simulink model "pmsm"  (R2021a)
settings: Solver=VariableStepAuto  StartTime=0.0  StopTime=5  RelTol=1e-3
values from neighbouring files (symbols this model uses):
  Fr = 5e-5    (= 5e-05)    [parame.m]
  J = 1.1e-3    (= 0.0011)    [parame.m]
  Ld = 1.8e-3    (= 0.0018)    [parame.m]
  Lq = 1.8e-3    (= 0.0018)    [parame.m]
  P = 2    [parame.m]
  Qf = 0.14    [parame.m]
  Rs = 0.76    [parame.m]
  Tmli = 1/fmli    (= 0.000333333333333)    [parame.m]
  Vdc = 220    [parame.m]
undefined symbols (not defined in the file or in its folder): sigbuilder_block
libraries: spsIGBTDiodeLib x6, spsVoltageMeasurementLib x3, spsDCVoltageSourceLib x1, simulink x1, spspowerguiLib x1
settings Model: Creator=21277  LastModifiedBy=PRO
settings SolverCC: AlgebraicLoopSolver=TrustRegion
settings OptimizationCC: LifeSpan=inf
settings DebuggingCC: UnconnectedInputMsg=none  UnconnectedOutputMsg=none  UnconnectedLineMsg=none  SFMachineParentedDataDiag=warning  ArithmeticOperatorsInVariantConditions=warning
settings ModelReferenceCC: EnableRefExpFcnMdlSchedulingChecks=off
settings SFSimCC: CustomCodeUndefinedFunction=UseInterfaceOnly
settings RTWCC: Description=Generic Real-Time Target
settings CodeAppCC: StateflowObjectComments=on

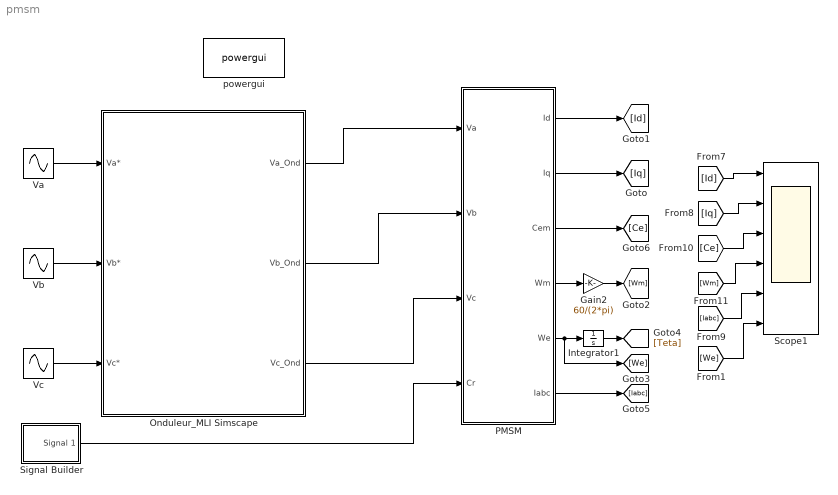
== system pmsm ==
  Gain2 : Gain  Gain=60/(2*pi)
  Integrator1 : Integrator
  Onduleur_MLI Simscape : Subsystem
  PMSM : Subsystem
  Scope1 : Scope  NumInputPorts=6
  Signal Builder : Subsystem  Tag=STV Subsys  LoadFcn=sigbuilder_block('load');  StartFcn=sigbuilder_block('start');  StopFcn=sigbuilder_block('stop');  ClipboardFcn=sigbuilder_block('clipboard');  mask(Sigbuilder block){tuvar=[0:10]}
      mask help: Simulink:masks:SigbuilderBlock_MD
      mask init:
      | if ~strcmp(get_param(bdroot(gcbh),'SimulationStatus'),'stopped') tuvar = sigbuilder_block('maskInit'); end
      settings: CopyFcn=sigbuilder_block('copy');  DeleteFcn=sigbuilder_block('delete');  ModelCloseFcn=sigbuilder_block('modelClose');  PreSaveFcn=sigbuilder_block('preSave');  PauseFcn=sigbuilder_block('pause');  ContinueFcn=sigbuilder_block('continue');  NameChangeFcn=sigbuilder_block('namechange');  OpenFcn=sigbuilder_block('open',[442.8 160.8 550.8 400.2 ]);  CloseFcn=sigbuilder_block('close');
      mask Display: plot(0, 0, 100, 100,[2, 2, 32, 32, 2], [68, 8, 8, 68, 68],[32, 2], [38, 38], [32, 19, 2],[53, 60, 44], [32, 17, 17, 2],[16, 16, 31, 31]);txt = getActiveGroup(gcbh);text(2, 100, txt,'verticalAlignment', 'top');
  Va : Sin  Amplitude=100  Frequency=50  SampleTime=0
  Vb : Sin  Amplitude=100  Frequency=50  Phase=-2*pi/3  SampleTime=0
  Vc : Sin  Amplitude=100  Frequency=50  Phase=2*pi/3  SampleTime=0
  powergui : spspowerguiLib/powergui  Priority=1  SimulationMode=Discrete  SampleTime=1e-5  frequency=60  Iterations=50  frequencyindice=0  Pbase=100e6  ErrMax=1e-4  UnitsV=kV  UnitsW=MW  buscounter=0  FunctionMessages=off  echomessages=off  EnableUseOfTLC=off  CurrentSourceSwitches=off  DisableSnubberDevices=off  DisableRonSwitches=off  DisableVfSwitches=off  DisplayEquations=off  AutomaticDiscreteSolvers=off  SolverType=Tustin/Backward Euler (TBE)  Interpol=off  ExternalGateDelay=off  methode=off  Ts=100  x0status=blocks  SPID=on  SwTol=0  HookPort=off  NonlinearTolerance=1e-4  nMaxIteration=100  ContinueOnMaxIteration=off  RestoreLinks=warning  ResistiveCurrentMeasurement=off  Frange=[0:2:500]  Ylog=off  Xlog=on  ShowGrid=off  save=off  variable=ZData  structure=0  ZoomFFT=off  StartTime=0.0  cycles=1  DisplayStyle=1  fundamental=60  FreqAxis=off  MaxFrequency=1000  frequencyindicesteady=1  RmsSteady=1  display=off
  wires:
  [Iabc] -> Scope1/5
  Signal Builder/1(Signal 1) -> PMSM/4(Cr)
  PMSM/6(Iabc) -> [Iabc]
  [Id] -> Scope1/1
  Gain2/1 -> [Wm]
  [Ce] -> Scope1/3
  [Iq] -> Scope1/2
  PMSM/1(Id) -> [Id]
  Onduleur_MLI Simscape/2(Vb_Ond) -> PMSM/2(Vb)
  [Wm] -> Scope1/4
  PMSM/5(We) -> Integrator1/1, [We]
  PMSM/2(Iq) -> [Iq]
  PMSM/4(Wm) -> Gain2/1
  Onduleur_MLI Simscape/3(Vc_Ond) -> PMSM/3(Vc)
  PMSM/3(Cem) -> [Ce]
  Onduleur_MLI Simscape/1(Va_Ond) -> PMSM/1(Va)
  Integrator1/1 -> [Teta]
  [We] -> Scope1/6
  Va/1 -> Onduleur_MLI Simscape/1(Va*)
  Vb/1 -> Onduleur_MLI Simscape/2(Vb*)
  Vc/1 -> Onduleur_MLI Simscape/3(Vc*)

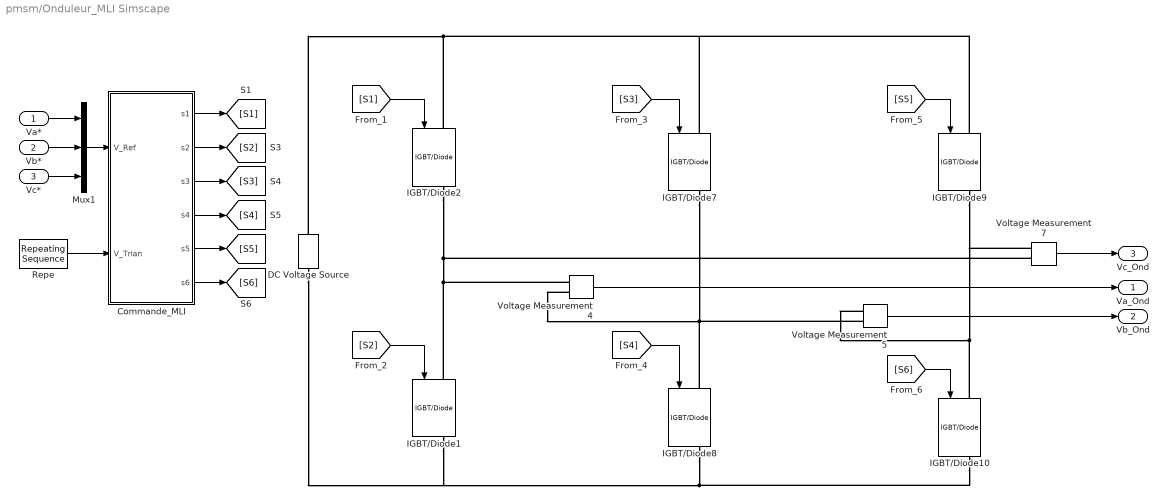
== system pmsm/Onduleur_MLI Simscape ==
  Va* : Inport
  Vb* : Inport  Port=2
  Vc* : Inport  Port=3
  Commande_MLI : Subsystem
  DC Voltage Source : spsDCVoltageSourceLib/DC Voltage Source  Amplitude=100  Measurements=None
  IGBT/Diode{1..2,7..10} (6 alike) : spsIGBTDiodeLib/IGBT//Diode  Ron=1e-3  Rs=1e5  Cs=inf  Measurements=on
  Mux1 : Mux  Inputs=3
  Repe : simulink/Sources/Repeating Sequence  rep_seq_t=[0 0.5 1]*Tmli  rep_seq_y=[-1 1 -1]*Vdc
  Voltage Measurement4 : spsVoltageMeasurementLib/Voltage Measurement  PhasorSimulation=off  OutputType=Complex  PSBequivalent=0
  Voltage Measurement5 : spsVoltageMeasurementLib/Voltage Measurement  PhasorSimulation=off  OutputType=Complex  PSBequivalent=0
  Voltage Measurement7 : spsVoltageMeasurementLib/Voltage Measurement  PhasorSimulation=off  OutputType=Complex  PSBequivalent=0
  Va_Ond : Outport
  Vb_Ond : Outport  Port=2
  Vc_Ond : Outport  Port=3
  wires:
  Voltage Measurement4/1 -> Va_Ond/1
  Voltage Measurement7/1 -> Vc_Ond/1
  Voltage Measurement5/1 -> Vb_Ond/1
  [S4] -> IGBT/Diode8/1
  Va*/1 -> Mux1/1
  [S5] -> IGBT/Diode9/1
  [S6] -> IGBT/Diode10/1
  Commande_MLI/3(s3) -> [S3]
  Commande_MLI/5(s5) -> [S5]
  [S3] -> IGBT/Diode7/1
  Vc*/1 -> Mux1/3
  Commande_MLI/2(s2) -> [S2]
  [S2] -> IGBT/Diode1/1
  Vb*/1 -> Mux1/2
  Commande_MLI/1(s1) -> [S1]
  [S1] -> IGBT/Diode2/1
  Mux1/1 -> Commande_MLI/1(V_Ref)
  Commande_MLI/6(s6) -> [S6]
  Repe/1 -> Commande_MLI/2(V_Trian)
  Commande_MLI/4(s4) -> [S4]
  connections:
  IGBT/Diode8/LConn1 -- Voltage Measurement4/LConn2 -- Voltage Measurement5/LConn1 -- IGBT/Diode7/RConn1
  IGBT/Diode2/LConn1 -- DC Voltage Source/RConn1 -- IGBT/Diode7/LConn1 -- IGBT/Diode9/LConn1
  IGBT/Diode10/RConn1 -- IGBT/Diode8/RConn1 -- DC Voltage Source/LConn1 -- IGBT/Diode1/RConn1
  IGBT/Diode10/LConn1 -- IGBT/Diode9/RConn1 -- Voltage Measurement7/LConn1 -- Voltage Measurement5/LConn2
  IGBT/Diode2/RConn1 -- Voltage Measurement7/LConn2 -- IGBT/Diode1/LConn1 -- Voltage Measurement4/LConn1

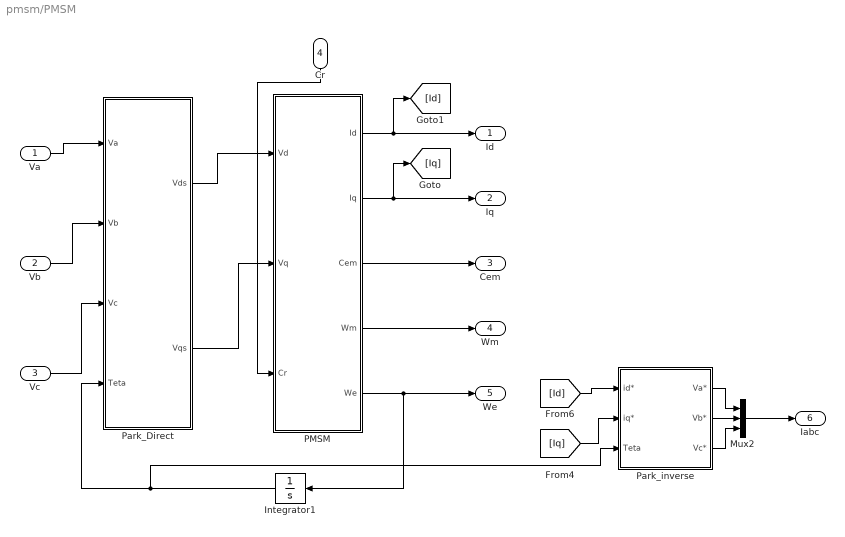
== system pmsm/PMSM ==
  Va : Inport
  Vb : Inport  Port=2
  Vc : Inport  Port=3
  Cr : Inport  Port=4
  Integrator1 : Integrator
  Mux2 : Mux  Inputs=3
  PMSM : Subsystem
  Park_Direct : Subsystem
  Park_inverse : Subsystem
  Id : Outport
  Iq : Outport  Port=2
  Cem : Outport  Port=3
  Wm : Outport  Port=4
  We : Outport  Port=5
  Iabc : Outport  Port=6
  wires:
  PMSM/5(We) -> Integrator1/1, We/1
  Park_Direct/2(Vqs) -> PMSM/2(Vq)
  Park_Direct/1(Vds) -> PMSM/1(Vd)
  PMSM/2(Iq) -> [Iq], Iq/1
  Cr/1 -> PMSM/3(Cr)
  Integrator1/1 -> Park_inverse/3(Teta), Park_Direct/4(Teta)
  PMSM/1(Id) -> [Id], Id/1
  Va/1 -> Park_Direct/1(Va)
  Vb/1 -> Park_Direct/2(Vb)
  PMSM/3(Cem) -> Cem/1
  Vc/1 -> Park_Direct/3(Vc)
  PMSM/4(Wm) -> Wm/1
  Park_inverse/1(Va*) -> Mux2/1
  Park_inverse/2(Vb*) -> Mux2/2
  Park_inverse/3(Vc*) -> Mux2/3
  [Iq] -> Park_inverse/2(iq*)
  Mux2/1 -> Iabc/1
  [Id] -> Park_inverse/1(id*)

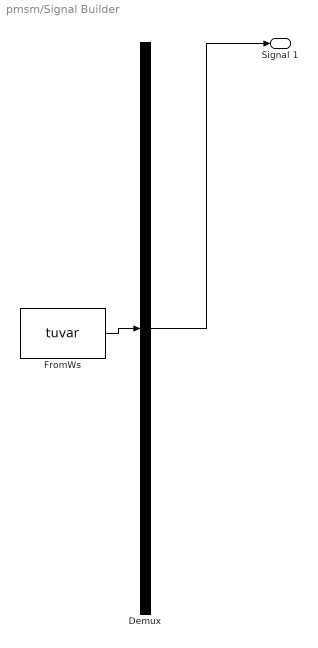
== system pmsm/Signal Builder ==
  Demux : Demux  Tag=STV Demux  Outputs=1
      settings: DisplayOption=none
  FromWs : FromWorkspace  Tag=STV FromWs  VariableName=tuvar
      SigBuilderData=|
      | common.afterFinalStr = 'Extrapolate'
      | common.sampleTime = 0
      | dataSet.timeRange = [0 1]
      | dataSet.name = 'Group 1'
      | sbobj.Groups.Name = 'Group 1'
      | sbobj.Groups.Signals.Name = 'Signal 1'
      | sbobj.Groups.Signals.XData = [0 0.1 0.1 0.3 0.3 0.6 0.6 1]
      | sbobj.Groups.Signals.YData = [0 0 10 10 5 5 0 0]
      | sbobj.Groups.TimeRange = [0 1]
  Signal 1 : Outport  Tag=STV Outport
  wires:
  FromWs/1 -> Demux/1
  Demux/1 -> Signal 1/1

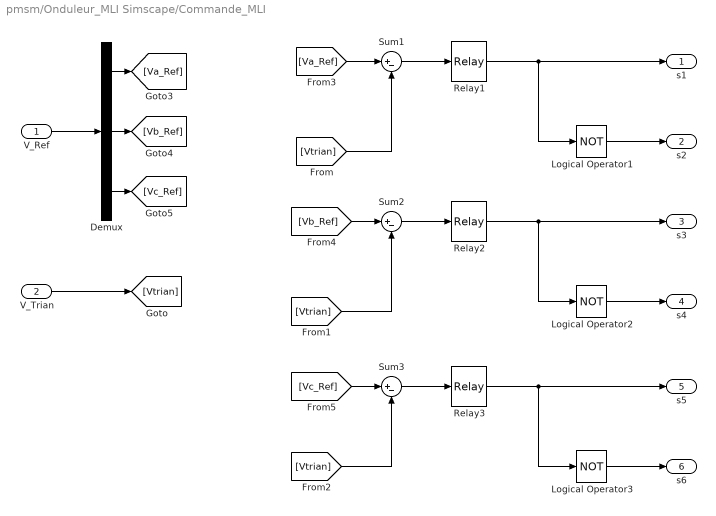
== system pmsm/Onduleur_MLI Simscape/Commande_MLI ==
  V_Ref : Inport
  V_Trian : Inport  Port=2
  Demux : Demux  Outputs=3
  Logical Operator1 : Logic  Operator=NOT  AllPortsSameDT=off  OutDataTypeStr=boolean
  Logical Operator2 : Logic  Operator=NOT  AllPortsSameDT=off  OutDataTypeStr=boolean
  Logical Operator3 : Logic  Operator=NOT  AllPortsSameDT=off  OutDataTypeStr=boolean
  Relay1 : Relay  OffSwitchValue=-eps
  Relay2 : Relay  OffSwitchValue=-eps
  Relay3 : Relay  OffSwitchValue=-eps
  Sum1 : Sum  Inputs=|+-
  Sum2 : Sum  Inputs=|+-
  Sum3 : Sum  Inputs=|+-
  s1 : Outport
  s2 : Outport  Port=2
  s3 : Outport  Port=3
  s4 : Outport  Port=4
  s5 : Outport  Port=5
  s6 : Outport  Port=6
  wires:
  Logical Operator2/1 -> s4/1
  Relay2/1 -> s3/1, Logical Operator2/1
  Sum2/1 -> Relay2/1
  V_Ref/1 -> Demux/1
  Relay1/1 -> s1/1, Logical Operator1/1
  Logical Operator1/1 -> s2/1
  Sum1/1 -> Relay1/1
  Sum3/1 -> Relay3/1
  Logical Operator3/1 -> s6/1
  Relay3/1 -> s5/1, Logical Operator3/1
  [Vtrian] -> Sum1/2
  [Vtrian] -> Sum2/2
  [Vtrian] -> Sum3/2
  [Va_Ref] -> Sum1/1
  [Vb_Ref] -> Sum2/1
  [Vc_Ref] -> Sum3/1
  Demux/1 -> [Va_Ref]
  Demux/2 -> [Vb_Ref]
  Demux/3 -> [Vc_Ref]
  V_Trian/1 -> [Vtrian]

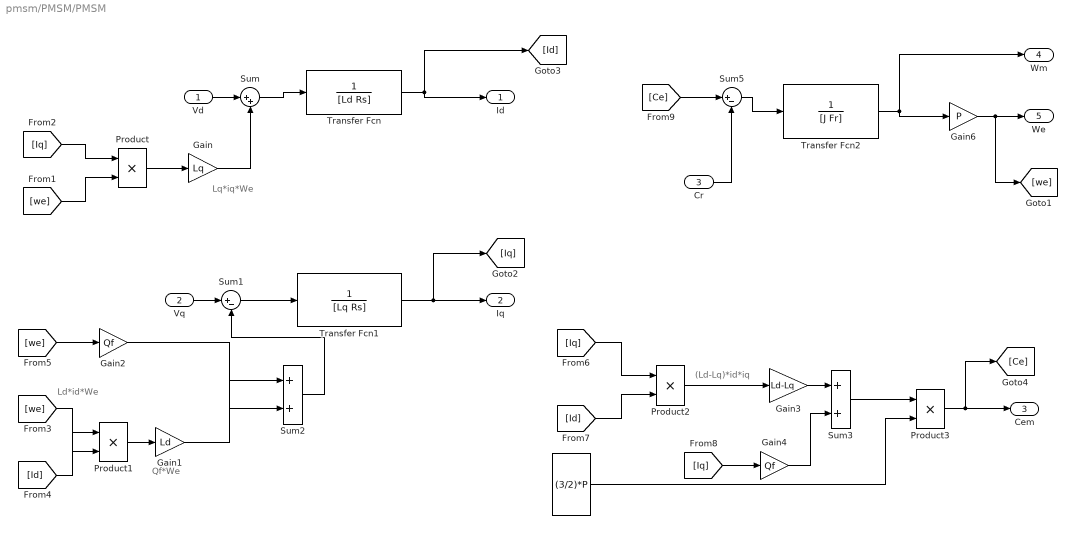
== system pmsm/PMSM/PMSM ==
  note: Lq*iq*We
  note: Ld*id*We
  note: Qf*We
  note: (Ld-Lq)*id*iq
  Vd : Inport
  Vq : Inport  Port=2
  Cr : Inport  Port=3
  " " : Constant  Value=(3/2)*P
  Gain : Gain  Gain=Lq
  Gain1 : Gain  Gain=Ld
  Gain2 : Gain  Gain=Qf
  Gain3 : Gain  Gain=Ld-Lq
  Gain4 : Gain  Gain=Qf
  Gain6 : Gain  Gain=P
  Product{,1..3} (4 alike) : Product
  Sum : Sum  Inputs=|++
  Sum1 : Sum  Inputs=|+-
  Sum2 : Sum
  Sum3 : Sum
  Sum5 : Sum  Inputs=|+-
  Transfer Fcn : TransferFcn  Denominator=[Ld Rs]
  Transfer Fcn1 : TransferFcn  Denominator=[Lq Rs]
  Transfer Fcn2 : TransferFcn  Denominator=[J Fr]
  Id : Outport
  Iq : Outport  Port=2
  Cem : Outport  Port=3
  Wm : Outport  Port=4
  We : Outport  Port=5
  wires:
  Vd/1 -> Sum/1
  Sum/1 -> Transfer Fcn/1
  Product/1 -> Gain/1
  [we] -> Product/2
  [Iq] -> Product/1
  Sum1/1 -> Transfer Fcn1/1
  Vq/1 -> Sum1/1
  Sum2/1 -> Sum1/2
  Transfer Fcn/1 -> Id/1, [Id]
  [we] -> Product1/2
  [Id] -> Product1/1
  Product1/1 -> Gain1/1
  Gain1/1 -> Sum2/1
  [we] -> Gain2/1
  Gain2/1 -> Sum2/2
  Transfer Fcn1/1 -> [Iq], Iq/1
  Product2/1 -> Gain3/1
  [Iq] -> Product2/1
  [Id] -> Product2/2
  Gain3/1 -> Sum3/1
  [Iq] -> Gain4/1
  Gain4/1 -> Sum3/2
  Sum3/1 -> Product3/1
  " "/1 -> Product3/2
  Product3/1 -> Cem/1, [Ce]
  Gain6/1 -> We/1, [we]
  [Ce] -> Sum5/1
  Cr/1 -> Sum5/2
  Sum5/1 -> Transfer Fcn2/1
  Transfer Fcn2/1 -> Gain6/1, Wm/1
  Gain/1 -> Sum/2

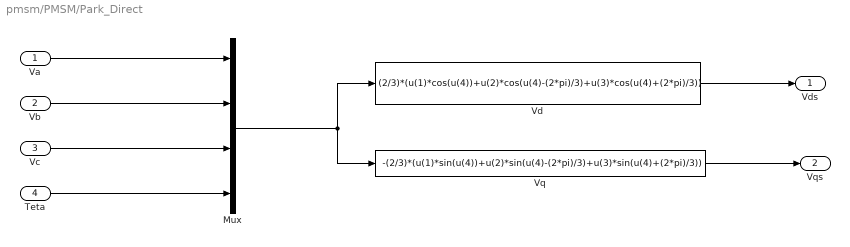
== system pmsm/PMSM/Park_Direct ==
  Va : Inport
  Vb : Inport  Port=2
  Vc : Inport  Port=3
  Teta : Inport  Port=4
  Mux : Mux
  Vd : Fcn  Expr=(2/3)*(u(1)*cos(u(4))+u(2)*cos(u(4)-(2*pi)/3)+u(3)*cos(u(4)+(2*pi)/3))
  Vq : Fcn  Expr=-(2/3)*(u(1)*sin(u(4))+u(2)*sin(u(4)-(2*pi)/3)+u(3)*sin(u(4)+(2*pi)/3))
  Vds : Outport
  Vqs : Outport  Port=2
  wires:
  Mux/1 -> Vq/1, Vd/1
  Vc/1 -> Mux/3
  Vb/1 -> Mux/2
  Vd/1 -> Vds/1
  Teta/1 -> Mux/4
  Va/1 -> Mux/1
  Vq/1 -> Vqs/1

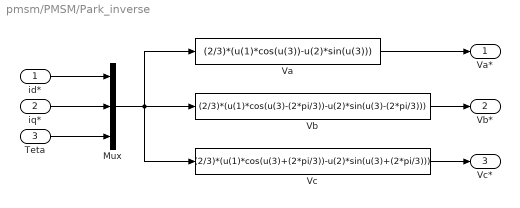
== system pmsm/PMSM/Park_inverse ==
  id* : Inport
  iq* : Inport  Port=2
  Teta : Inport  Port=3
  Mux : Mux  Inputs=3
  Va : Fcn  Expr=(2/3)*(u(1)*cos(u(3))-u(2)*sin(u(3)))
  Vb : Fcn  Expr=(2/3)*(u(1)*cos(u(3)-(2*pi/3))-u(2)*sin(u(3)-(2*pi/3)))
  Vc : Fcn  Expr=(2/3)*(u(1)*cos(u(3)+(2*pi/3))-u(2)*sin(u(3)+(2*pi/3)))
  Va* : Outport
  Vb* : Outport  Port=2
  Vc* : Outport  Port=3
  wires:
  Vb/1 -> Vb*/1
  Teta/1 -> Mux/3
  iq*/1 -> Mux/2
  Vc/1 -> Vc*/1
  Mux/1 -> Vc/1, Vb/1, Va/1
  Va/1 -> Va*/1
  id*/1 -> Mux/1
